simulink model "sim_part2"  (R2022b)
settings: Solver=VariableStepAuto  StartTime=0.0  StopTime=25  RelTol=1e-3
undefined symbols (not defined in the file): matA1, matB1
libraries: cstblocks x1
settings Model: Creator=alon  LastModifiedBy=binya
settings SolverCC: AlgebraicLoopSolver=TrustRegion
settings DebuggingCC: UnconnectedInputMsg=warning  UnconnectedOutputMsg=warning  UnconnectedLineMsg=warning  SFMachineParentedDataDiag=warning
settings ModelReferenceCC: EnableRefExpFcnMdlSchedulingChecks=on

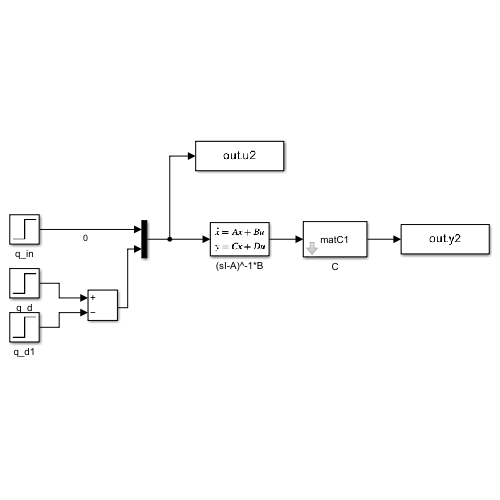
[thumbnail: Simulink's stored preview of the top-level diagram]
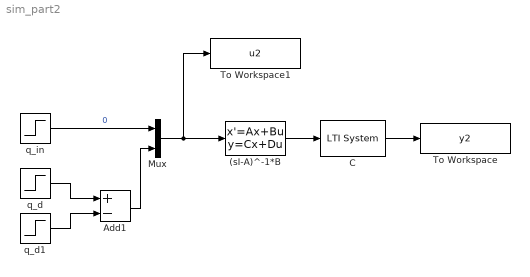
== system sim_part2 ==
  (sI-A)^-1*B : StateSpace  A=matA1  B=matB1  C=eye(3)  D=[[0 0];[0 0];[0 0]]  InitialCondition=0
  Add1 : Sum  Inputs=+-
  C : cstblocks/LTI System  sys=matC1  IC=[]
  Mux : Mux  Inputs=2
  To Workspace : ToWorkspace  VariableName=y2  SaveFormat=Timeseries  SampleTime=-1
  To Workspace1 : ToWorkspace  VariableName=u2  SaveFormat=Timeseries  SampleTime=-1
  q_d : Step  Time=0  After=12  SampleTime=0
  q_d1 : Step  Time=2.3  After=12  SampleTime=0
  q_in : Step  Time=0  After=0  SampleTime=0
  wires:
  Mux/1 -> To Workspace1/1, (sI-A)^-1*B/1
  q_d/1 -> Add1/1
  Add1/1 -> Mux/2
  q_d1/1 -> Add1/2
  q_in/1 -> Mux/1  "0"
  C/1 -> To Workspace/1
  (sI-A)^-1*B/1 -> C/1
